simulink model "kiem_chung_xe_day"  (R2025a)
settings: Solver=VariableStepAuto  StartTime=0.0  StopTime=1  RelTol=1e-3
values from neighbouring files (symbols this model uses):
  Kdx = 159.386436554    [PID_xe_day.mat]
  Kix = 25638.0154538    [PID_xe_day.mat]
  Kpx = 2786.27563751    [PID_xe_day.mat]
undefined symbols (not defined in the file or in its folder): G1
settings Model: SimulationMode=accelerator  Creator=datng  LastModifiedBy=datng

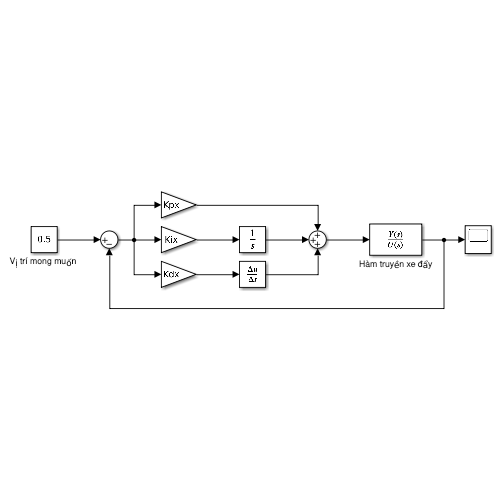
[thumbnail: Simulink's stored preview of the top-level diagram]
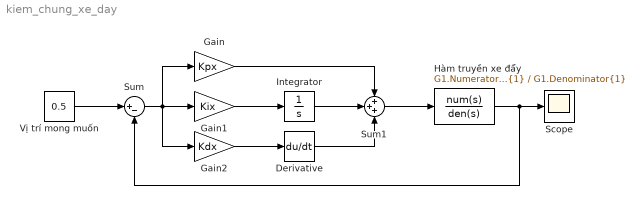
== system kiem_chung_xe_day ==
  Derivative : Derivative  CoefficientInTFapproximation=0
  Gain : Gain  Gain=Kpx
  Gain1 : Gain  Gain=Kix
  Gain2 : Gain  Gain=Kdx
  Hàm truyền xe đẩy : TransferFcn  Numerator=G1.Numerator{1}  Denominator=G1.Denominator{1}
  Integrator : Integrator
  Scope : Scope
      settings: ActiveDisplayYMinimum=-0.079116046223831019  ActiveDisplayYMaximum=0.71204441601447932  YLabel=x (m)
  Sum : Sum  Inputs=|+-
  Sum1 : Sum  Inputs=+++
  "Vị trí mong muốn " : Constant  Value=0.5
  wires:
  "Vị trí mong muốn "/1 -> Sum/1
  Sum/1 -> Gain/1, Gain2/1, Gain1/1
  Gain1/1 -> Integrator/1
  Integrator/1 -> Sum1/2
  Derivative/1 -> Sum1/3
  Gain2/1 -> Derivative/1
  Gain/1 -> Sum1/1
  Sum1/1 -> Hàm truyền xe đẩy/1
  Hàm truyền xe đẩy/1 -> Scope/1, Sum/2
